simulink model "c10mfode2"  (R2017a)
settings: Solver=ode15s  StartTime=0.0  StopTime=4  RelTol=1e-9  EnableMultiTasking=on
PreLoadFcn:
  | ww=[1e-3 1e3]; n=9;
undefined symbols (not defined in the file): N
settings Model: Creator=yj  LastModifiedBy=Professor Dingyu Xue
settings DataIOCC: SaveFormat=Array  SignalLoggingSaveFormat=ModelDataLogs  SignalLoggingName=sigsOut
settings OptimizationCC: ExpressionDepthLimit=2147483647  InitFltsAndDblsToZero=on  LifeSpan=inf
settings DebuggingCC: SaveWithParameterizedLinksMsg=none  UnderspecifiedInitializationDetection=Classic  MergeDetectMultiDrivingBlocksExec=none  SignalResolutionControl=TryResolveAllWithWarning  MultiTaskDSMMsg=warning  MultiTaskCondExecSysMsg=none  FcnCallInpInsideContextMsg=warning  StateNameClashWarn=warning  SFUnexpectedBacktrackingDiag=warning  SFNoUnconditionalDefaultTransitionDiag=warning  SFExecutionAtInitializationDiag=none
settings HardwareCC: ProdBitPerPointer=32  ProdBitPerSizeT=32  ProdBitPerPtrDiffT=32  ProdLargestAtomicFloat=None  ProdIntDivRoundTo=Undefined  ProdEndianess=Unspecified  ProdWordSize=32  ProdHWDeviceType=32-bit Generic  TargetUnknown=on
settings ModelReferenceCC: PropagateSignalLabelsOutOfModel=off
settings GRTTargetCC: TargetLangStandard=C89/C90 (ANSI)  CombineOutputUpdateFcns=off  GRTInterface=on
settings ConfigComp: CovMetricSettings=dw  CovHtmlReporting=on  CovSaveCumulativeToWorkspaceVar=on  CovSaveSingleToWorkspaceVar=on  CovExternalEMLEnable=off

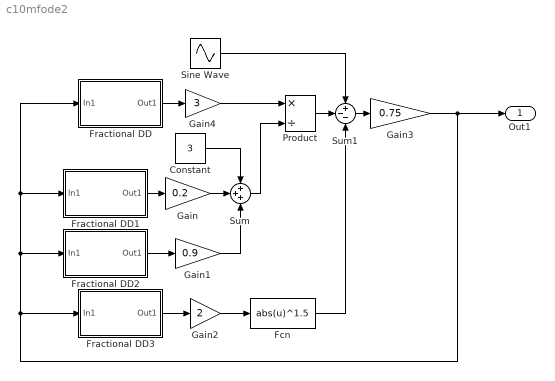
== system c10mfode2 ==
  Constant : Constant  Value=3
  Fcn : Fcn  Expr=abs(u)^1.5
  Fractional DD : Subsystem  mask{gam=0.9, ww=ww, n=N}
      mask prompts: gam "Derivative order gamma"; ww "Frequency range [wb,wh]"; n "Apprixmation order"
      mask init:
      | wb=ww(1); wh=ww(2); G=ousta_fod(gam,n,wb,wh);
      | num=G.num{1}; den=G.den{1}; T=1/wh; str='Fractional\n';
      | if isnumeric(gam)
      | 	if gam>0, str=[str, 'Der  s^' num2str(gam) ];
      | 	else, str=[str, 'Int  s^{' num2str(gam) '}']; end
      | else, str=[str, 'Der  s^gam']; end
      mask Display: disp(str)
  Fractional DD1 : Subsystem  mask{gam=0.8, ww=ww, n=N}
      mask prompts: gam "Derivative order gamma"; ww "Frequency range [wb,wh]"; n "Apprixmation order"
      mask init: same as c10mfode2/Fractional DD
      mask Display: disp(str)
  Fractional DD2 : Subsystem  mask{gam=0.2, ww=ww, n=N}
      mask prompts: gam "Derivative order gamma"; ww "Frequency range [wb,wh]"; n "Apprixmation order"
      mask init: same as c10mfode2/Fractional DD
      mask Display: disp(str)
  Fractional DD3 : Subsystem  mask{gam=0.7, ww=ww, n=N}
      mask prompts: gam "Derivative order gamma"; ww "Frequency range [wb,wh]"; n "Apprixmation order"
      mask init: same as c10mfode2/Fractional DD
      mask Display: disp(str)
  Gain : Gain  Gain=0.2  SaturateOnIntegerOverflow=on  OutDataTypeStr=Inherit: Same as input  ParamDataTypeStr=Inherit: Same as input
  Gain1 : Gain  Gain=0.9  SaturateOnIntegerOverflow=on  OutDataTypeStr=Inherit: Same as input  ParamDataTypeStr=Inherit: Same as input
  Gain2 : Gain  Gain=2  SaturateOnIntegerOverflow=on  OutDataTypeStr=Inherit: Same as input  ParamDataTypeStr=Inherit: Same as input
  Gain3 : Gain  Gain=0.75  SaturateOnIntegerOverflow=on  OutDataTypeStr=Inherit: Same as input  ParamDataTypeStr=Inherit: Same as input
  Gain4 : Gain  Gain=3  SaturateOnIntegerOverflow=on  OutDataTypeStr=Inherit: Same as input  ParamDataTypeStr=Inherit: Same as input
  Product : Product  Inputs=*/  SaturateOnIntegerOverflow=on  OutDataTypeStr=Inherit: Same as first input
  Sine Wave : Sin  Amplitude=5  Frequency=20  SampleTime=0
  Sum : Sum  Inputs=+++  SaturateOnIntegerOverflow=on
  Sum1 : Sum  Inputs=+--  SaturateOnIntegerOverflow=on
  Out1 : Outport
  wires:
  Fractional DD2/1(Out1) -> Gain1/1
  Fractional DD/1(Out1) -> Gain4/1
  Sum/1 -> Product/2
  Fractional DD3/1(Out1) -> Gain2/1
  Sine Wave/1 -> Sum1/1
  Product/1 -> Sum1/2
  Sum1/1 -> Gain3/1
  Gain/1 -> Sum/2
  Gain1/1 -> Sum/3
  Constant/1 -> Sum/1
  Gain4/1 -> Product/1
  Gain2/1 -> Fcn/1
  Fcn/1 -> Sum1/3
  Fractional DD1/1(Out1) -> Gain/1
  Gain3/1 -> Fractional DD3/1(In1), Fractional DD2/1(In1), Fractional DD1/1(In1), Fractional DD/1(In1), Out1/1

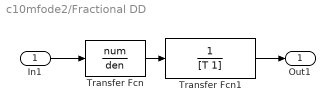
== system c10mfode2/Fractional DD ==
  In1 : Inport
  Transfer Fcn : TransferFcn  Numerator=num  Denominator=den
  Transfer Fcn1 : TransferFcn  Numerator=1  Denominator=[T 1]
  Out1 : Outport
  wires:
  In1/1 -> Transfer Fcn/1
  Transfer Fcn/1 -> Transfer Fcn1/1
  Transfer Fcn1/1 -> Out1/1

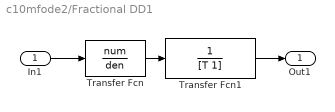
== system c10mfode2/Fractional DD1 ==
  In1 : Inport
  Transfer Fcn : TransferFcn  Numerator=num  Denominator=den
  Transfer Fcn1 : TransferFcn  Numerator=1  Denominator=[T 1]
  Out1 : Outport
  wires:
  Transfer Fcn1/1 -> Out1/1
  Transfer Fcn/1 -> Transfer Fcn1/1
  In1/1 -> Transfer Fcn/1

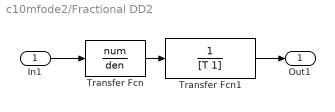
== system c10mfode2/Fractional DD2 ==
  In1 : Inport
  Transfer Fcn : TransferFcn  Numerator=num  Denominator=den
  Transfer Fcn1 : TransferFcn  Numerator=1  Denominator=[T 1]
  Out1 : Outport
  wires:
  In1/1 -> Transfer Fcn/1
  Transfer Fcn/1 -> Transfer Fcn1/1
  Transfer Fcn1/1 -> Out1/1

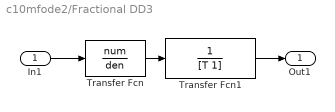
== system c10mfode2/Fractional DD3 ==
  In1 : Inport
  Transfer Fcn : TransferFcn  Numerator=num  Denominator=den
  Transfer Fcn1 : TransferFcn  Numerator=1  Denominator=[T 1]
  Out1 : Outport
  wires:
  Transfer Fcn1/1 -> Out1/1
  Transfer Fcn/1 -> Transfer Fcn1/1
  In1/1 -> Transfer Fcn/1
